simulink model "check_fence"  (Simulink 7.4)
settings: Solver=ode45  StartTime=0.0  StopTime=10.0  RelTol=1e-3
libraries: xbsIndex_r4 x293
(part 2 of 2)

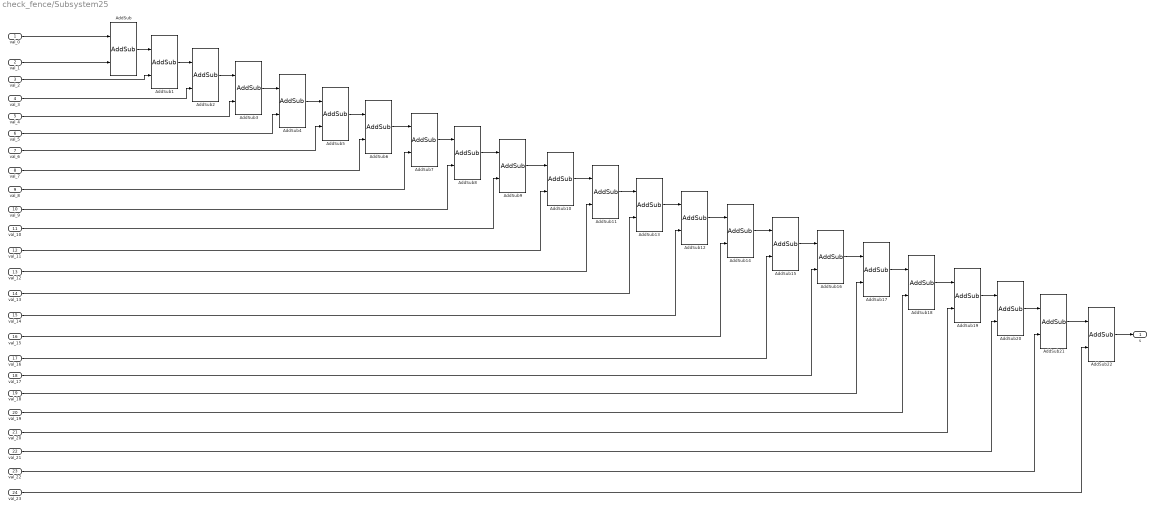
== system check_fence/Subsystem25 ==
  val_0 : Inport
  val_1 : Inport  Port=2
  val_2 : Inport  Port=3
  val_3 : Inport  Port=4
  val_4 : Inport  Port=5
  val_5 : Inport  Port=6
  val_6 : Inport  Port=7
  val_7 : Inport  Port=8
  val_8 : Inport  Port=9
  val_9 : Inport  Port=10
  val_10 : Inport  Port=11
  val_11 : Inport  Port=12
  val_12 : Inport  Port=13
  val_13 : Inport  Port=14
  val_14 : Inport  Port=15
  val_15 : Inport  Port=16
  val_16 : Inport  Port=17
  val_17 : Inport  Port=18
  val_18 : Inport  Port=19
  val_19 : Inport  Port=20
  val_20 : Inport  Port=21
  val_21 : Inport  Port=22
  val_22 : Inport  Port=23
  val_23 : Inport  Port=24
  AddSub{,1..22} (23 alike) : xbsIndex_r4/AddSub  mode=Addition  use_carryin=off  use_carryout=off  en=off  latency=0  precision=Full  arith_type=Unsigned  n_bits=16  bin_pt=14  quantization=Truncate  overflow=Wrap  dbl_ovrd=off  use_behavioral_HDL=off  hw_selection=Fabric  pipelined=off  block_type=addsub
  s : Outport
  wires:
  val_23/1 -> AddSub22/2
  val_22/1 -> AddSub21/2
  val_21/1 -> AddSub20/2
  val_20/1 -> AddSub19/2
  val_19/1 -> AddSub18/2
  val_18/1 -> AddSub17/2
  val_17/1 -> AddSub16/2
  val_16/1 -> AddSub15/2
  val_15/1 -> AddSub14/2
  val_14/1 -> AddSub12/2
  val_13/1 -> AddSub13/2
  val_12/1 -> AddSub11/2
  val_11/1 -> AddSub10/2
  val_10/1 -> AddSub9/2
  val_9/1 -> AddSub8/2
  val_8/1 -> AddSub7/2
  val_7/1 -> AddSub6/2
  val_6/1 -> AddSub5/2
  val_5/1 -> AddSub4/2
  val_4/1 -> AddSub3/2
  val_3/1 -> AddSub2/2
  val_2/1 -> AddSub1/2
  AddSub22/1 -> s/1
  AddSub21/1 -> AddSub22/1
  AddSub20/1 -> AddSub21/1
  AddSub19/1 -> AddSub20/1
  AddSub18/1 -> AddSub19/1
  AddSub17/1 -> AddSub18/1
  AddSub16/1 -> AddSub17/1
  AddSub15/1 -> AddSub16/1
  AddSub14/1 -> AddSub15/1
  AddSub12/1 -> AddSub14/1
  AddSub13/1 -> AddSub12/1
  AddSub11/1 -> AddSub13/1
  AddSub10/1 -> AddSub11/1
  AddSub9/1 -> AddSub10/1
  AddSub8/1 -> AddSub9/1
  AddSub7/1 -> AddSub8/1
  AddSub6/1 -> AddSub7/1
  AddSub5/1 -> AddSub6/1
  AddSub4/1 -> AddSub5/1
  AddSub3/1 -> AddSub4/1
  AddSub2/1 -> AddSub3/1
  AddSub1/1 -> AddSub2/1
  AddSub/1 -> AddSub1/1
  val_1/1 -> AddSub/2
  val_0/1 -> AddSub/1

== system check_fence/Subsystem3 ==
  warp_reg_addr : Inport
  warp_id : Inport  Port=2
  cta_id_in : Inport  Port=3
  cta_ld_en : Inport  Port=4
  is_fenced_in : Inport  Port=5
  is_fenced_ld_en : Inport  Port=6
  Constant : xbsIndex_r4/Constant  arith_type=Boolean  const=0  n_bits=16  bin_pt=14  explicit_period=off  period=1  equ=P=C  opselect=C  inp2=PCIN>>17  opr=+  inp1=P  carry=CIN  dbl_ovrd=off  block_type=constant
  Constant1 : xbsIndex_r4/Constant  arith_type=Boolean  const=0  n_bits=16  bin_pt=14  explicit_period=off  period=1  equ=P=C  opselect=C  inp2=PCIN>>17  opr=+  inp1=P  carry=CIN  dbl_ovrd=off  block_type=constant
  Constant2 : xbsIndex_r4/Constant  arith_type=Unsigned  const=0  n_bits=1  bin_pt=0  explicit_period=off  period=1  equ=P=C  opselect=C  inp2=PCIN>>17  opr=+  inp1=P  carry=CIN  dbl_ovrd=off  block_type=constant
  Mux : xbsIndex_r4/Mux  inputs=2  en=off  latency=0  precision=Full  arith_type=Unsigned  n_bits=16  bin_pt=14  quantization=Truncate  overflow=Wrap  dbl_ovrd=off  block_type=mux
  Mux1 : xbsIndex_r4/Mux  inputs=2  en=off  latency=0  precision=Full  arith_type=Unsigned  n_bits=16  bin_pt=14  quantization=Truncate  overflow=Wrap  dbl_ovrd=off  block_type=mux
  Mux2 : xbsIndex_r4/Mux  inputs=2  en=off  latency=0  precision=Full  arith_type=Unsigned  n_bits=16  bin_pt=14  quantization=Truncate  overflow=Wrap  dbl_ovrd=off  block_type=mux
  Register : xbsIndex_r4/Register  init=0  rst=off  en=on  dbl_ovrd=off  block_type=register
  Register1 : xbsIndex_r4/Register  init=0  rst=off  en=on  dbl_ovrd=off  block_type=register
  Relational : xbsIndex_r4/Relational  mode=a=b  en=off  latency=0  dbl_ovrd=off  block_type=relational
  Relational1 : xbsIndex_r4/Relational  mode=a=b  en=off  latency=0  dbl_ovrd=off  block_type=relational
  is_fenced_out : Outport
  data_valid : Outport  Port=2
  wires:
  cta_id_in/1 -> Register/1, Relational1/1
  is_fenced_in/1 -> Register1/1
  warp_reg_addr/1 -> Relational/1
  warp_id/1 -> Relational/2
  Mux/1 -> Register/2
  cta_ld_en/1 -> Mux/3
  Constant/1 -> Mux/2
  Relational/1 -> Mux/1, Mux1/1
  Mux1/1 -> Register1/2
  is_fenced_ld_en/1 -> Mux1/3
  Constant1/1 -> Mux1/2
  Relational1/1 -> Mux2/1, data_valid/1
  Constant2/1 -> Mux2/2
  Register/1 -> Relational1/2
  Register1/1 -> Mux2/3
  Mux2/1 -> is_fenced_out/1

== system check_fence/Subsystem4 ==
  warp_reg_addr : Inport
  warp_id : Inport  Port=2
  cta_id_in : Inport  Port=3
  cta_ld_en : Inport  Port=4
  is_fenced_in : Inport  Port=5
  is_fenced_ld_en : Inport  Port=6
  Constant : xbsIndex_r4/Constant  arith_type=Boolean  const=0  n_bits=16  bin_pt=14  explicit_period=off  period=1  equ=P=C  opselect=C  inp2=PCIN>>17  opr=+  inp1=P  carry=CIN  dbl_ovrd=off  block_type=constant
  Constant1 : xbsIndex_r4/Constant  arith_type=Boolean  const=0  n_bits=16  bin_pt=14  explicit_period=off  period=1  equ=P=C  opselect=C  inp2=PCIN>>17  opr=+  inp1=P  carry=CIN  dbl_ovrd=off  block_type=constant
  Constant2 : xbsIndex_r4/Constant  arith_type=Unsigned  const=0  n_bits=1  bin_pt=0  explicit_period=off  period=1  equ=P=C  opselect=C  inp2=PCIN>>17  opr=+  inp1=P  carry=CIN  dbl_ovrd=off  block_type=constant
  Mux : xbsIndex_r4/Mux  inputs=2  en=off  latency=0  precision=Full  arith_type=Unsigned  n_bits=16  bin_pt=14  quantization=Truncate  overflow=Wrap  dbl_ovrd=off  block_type=mux
  Mux1 : xbsIndex_r4/Mux  inputs=2  en=off  latency=0  precision=Full  arith_type=Unsigned  n_bits=16  bin_pt=14  quantization=Truncate  overflow=Wrap  dbl_ovrd=off  block_type=mux
  Mux2 : xbsIndex_r4/Mux  inputs=2  en=off  latency=0  precision=Full  arith_type=Unsigned  n_bits=16  bin_pt=14  quantization=Truncate  overflow=Wrap  dbl_ovrd=off  block_type=mux
  Register : xbsIndex_r4/Register  init=0  rst=off  en=on  dbl_ovrd=off  block_type=register
  Register1 : xbsIndex_r4/Register  init=0  rst=off  en=on  dbl_ovrd=off  block_type=register
  Relational : xbsIndex_r4/Relational  mode=a=b  en=off  latency=0  dbl_ovrd=off  block_type=relational
  Relational1 : xbsIndex_r4/Relational  mode=a=b  en=off  latency=0  dbl_ovrd=off  block_type=relational
  is_fenced_out : Outport
  data_valid : Outport  Port=2
  wires:
  Mux2/1 -> is_fenced_out/1
  Register1/1 -> Mux2/3
  Register/1 -> Relational1/2
  Constant2/1 -> Mux2/2
  Relational1/1 -> data_valid/1, Mux2/1
  Constant1/1 -> Mux1/2
  is_fenced_ld_en/1 -> Mux1/3
  Mux1/1 -> Register1/2
  Relational/1 -> Mux1/1, Mux/1
  Constant/1 -> Mux/2
  cta_ld_en/1 -> Mux/3
  Mux/1 -> Register/2
  warp_id/1 -> Relational/2
  warp_reg_addr/1 -> Relational/1
  is_fenced_in/1 -> Register1/1
  cta_id_in/1 -> Relational1/1, Register/1

== system check_fence/Subsystem5 ==
  warp_reg_addr : Inport
  warp_id : Inport  Port=2
  cta_id_in : Inport  Port=3
  cta_ld_en : Inport  Port=4
  is_fenced_in : Inport  Port=5
  is_fenced_ld_en : Inport  Port=6
  Constant : xbsIndex_r4/Constant  arith_type=Boolean  const=0  n_bits=16  bin_pt=14  explicit_period=off  period=1  equ=P=C  opselect=C  inp2=PCIN>>17  opr=+  inp1=P  carry=CIN  dbl_ovrd=off  block_type=constant
  Constant1 : xbsIndex_r4/Constant  arith_type=Boolean  const=0  n_bits=16  bin_pt=14  explicit_period=off  period=1  equ=P=C  opselect=C  inp2=PCIN>>17  opr=+  inp1=P  carry=CIN  dbl_ovrd=off  block_type=constant
  Constant2 : xbsIndex_r4/Constant  arith_type=Unsigned  const=0  n_bits=1  bin_pt=0  explicit_period=off  period=1  equ=P=C  opselect=C  inp2=PCIN>>17  opr=+  inp1=P  carry=CIN  dbl_ovrd=off  block_type=constant
  Mux : xbsIndex_r4/Mux  inputs=2  en=off  latency=0  precision=Full  arith_type=Unsigned  n_bits=16  bin_pt=14  quantization=Truncate  overflow=Wrap  dbl_ovrd=off  block_type=mux
  Mux1 : xbsIndex_r4/Mux  inputs=2  en=off  latency=0  precision=Full  arith_type=Unsigned  n_bits=16  bin_pt=14  quantization=Truncate  overflow=Wrap  dbl_ovrd=off  block_type=mux
  Mux2 : xbsIndex_r4/Mux  inputs=2  en=off  latency=0  precision=Full  arith_type=Unsigned  n_bits=16  bin_pt=14  quantization=Truncate  overflow=Wrap  dbl_ovrd=off  block_type=mux
  Register : xbsIndex_r4/Register  init=0  rst=off  en=on  dbl_ovrd=off  block_type=register
  Register1 : xbsIndex_r4/Register  init=0  rst=off  en=on  dbl_ovrd=off  block_type=register
  Relational : xbsIndex_r4/Relational  mode=a=b  en=off  latency=0  dbl_ovrd=off  block_type=relational
  Relational1 : xbsIndex_r4/Relational  mode=a=b  en=off  latency=0  dbl_ovrd=off  block_type=relational
  is_fenced_out : Outport
  data_valid : Outport  Port=2
  wires:
  cta_id_in/1 -> Register/1, Relational1/1
  is_fenced_in/1 -> Register1/1
  warp_reg_addr/1 -> Relational/1
  warp_id/1 -> Relational/2
  Mux/1 -> Register/2
  cta_ld_en/1 -> Mux/3
  Constant/1 -> Mux/2
  Relational/1 -> Mux/1, Mux1/1
  Mux1/1 -> Register1/2
  is_fenced_ld_en/1 -> Mux1/3
  Constant1/1 -> Mux1/2
  Relational1/1 -> Mux2/1, data_valid/1
  Constant2/1 -> Mux2/2
  Register/1 -> Relational1/2
  Register1/1 -> Mux2/3
  Mux2/1 -> is_fenced_out/1

== system check_fence/Subsystem6 ==
  warp_reg_addr : Inport
  warp_id : Inport  Port=2
  cta_id_in : Inport  Port=3
  cta_ld_en : Inport  Port=4
  is_fenced_in : Inport  Port=5
  is_fenced_ld_en : Inport  Port=6
  Constant : xbsIndex_r4/Constant  arith_type=Boolean  const=0  n_bits=16  bin_pt=14  explicit_period=off  period=1  equ=P=C  opselect=C  inp2=PCIN>>17  opr=+  inp1=P  carry=CIN  dbl_ovrd=off  block_type=constant
  Constant1 : xbsIndex_r4/Constant  arith_type=Boolean  const=0  n_bits=16  bin_pt=14  explicit_period=off  period=1  equ=P=C  opselect=C  inp2=PCIN>>17  opr=+  inp1=P  carry=CIN  dbl_ovrd=off  block_type=constant
  Constant2 : xbsIndex_r4/Constant  arith_type=Unsigned  const=0  n_bits=1  bin_pt=0  explicit_period=off  period=1  equ=P=C  opselect=C  inp2=PCIN>>17  opr=+  inp1=P  carry=CIN  dbl_ovrd=off  block_type=constant
  Mux : xbsIndex_r4/Mux  inputs=2  en=off  latency=0  precision=Full  arith_type=Unsigned  n_bits=16  bin_pt=14  quantization=Truncate  overflow=Wrap  dbl_ovrd=off  block_type=mux
  Mux1 : xbsIndex_r4/Mux  inputs=2  en=off  latency=0  precision=Full  arith_type=Unsigned  n_bits=16  bin_pt=14  quantization=Truncate  overflow=Wrap  dbl_ovrd=off  block_type=mux
  Mux2 : xbsIndex_r4/Mux  inputs=2  en=off  latency=0  precision=Full  arith_type=Unsigned  n_bits=16  bin_pt=14  quantization=Truncate  overflow=Wrap  dbl_ovrd=off  block_type=mux
  Register : xbsIndex_r4/Register  init=0  rst=off  en=on  dbl_ovrd=off  block_type=register
  Register1 : xbsIndex_r4/Register  init=0  rst=off  en=on  dbl_ovrd=off  block_type=register
  Relational : xbsIndex_r4/Relational  mode=a=b  en=off  latency=0  dbl_ovrd=off  block_type=relational
  Relational1 : xbsIndex_r4/Relational  mode=a=b  en=off  latency=0  dbl_ovrd=off  block_type=relational
  is_fenced_out : Outport
  data_valid : Outport  Port=2
  wires:
  Mux2/1 -> is_fenced_out/1
  Register1/1 -> Mux2/3
  Register/1 -> Relational1/2
  Constant2/1 -> Mux2/2
  Relational1/1 -> data_valid/1, Mux2/1
  Constant1/1 -> Mux1/2
  is_fenced_ld_en/1 -> Mux1/3
  Mux1/1 -> Register1/2
  Relational/1 -> Mux1/1, Mux/1
  Constant/1 -> Mux/2
  cta_ld_en/1 -> Mux/3
  Mux/1 -> Register/2
  warp_id/1 -> Relational/2
  warp_reg_addr/1 -> Relational/1
  is_fenced_in/1 -> Register1/1
  cta_id_in/1 -> Relational1/1, Register/1

== system check_fence/Subsystem7 ==
  warp_reg_addr : Inport
  warp_id : Inport  Port=2
  cta_id_in : Inport  Port=3
  cta_ld_en : Inport  Port=4
  is_fenced_in : Inport  Port=5
  is_fenced_ld_en : Inport  Port=6
  Constant : xbsIndex_r4/Constant  arith_type=Boolean  const=0  n_bits=16  bin_pt=14  explicit_period=off  period=1  equ=P=C  opselect=C  inp2=PCIN>>17  opr=+  inp1=P  carry=CIN  dbl_ovrd=off  block_type=constant
  Constant1 : xbsIndex_r4/Constant  arith_type=Boolean  const=0  n_bits=16  bin_pt=14  explicit_period=off  period=1  equ=P=C  opselect=C  inp2=PCIN>>17  opr=+  inp1=P  carry=CIN  dbl_ovrd=off  block_type=constant
  Constant2 : xbsIndex_r4/Constant  arith_type=Unsigned  const=0  n_bits=1  bin_pt=0  explicit_period=off  period=1  equ=P=C  opselect=C  inp2=PCIN>>17  opr=+  inp1=P  carry=CIN  dbl_ovrd=off  block_type=constant
  Mux : xbsIndex_r4/Mux  inputs=2  en=off  latency=0  precision=Full  arith_type=Unsigned  n_bits=16  bin_pt=14  quantization=Truncate  overflow=Wrap  dbl_ovrd=off  block_type=mux
  Mux1 : xbsIndex_r4/Mux  inputs=2  en=off  latency=0  precision=Full  arith_type=Unsigned  n_bits=16  bin_pt=14  quantization=Truncate  overflow=Wrap  dbl_ovrd=off  block_type=mux
  Mux2 : xbsIndex_r4/Mux  inputs=2  en=off  latency=0  precision=Full  arith_type=Unsigned  n_bits=16  bin_pt=14  quantization=Truncate  overflow=Wrap  dbl_ovrd=off  block_type=mux
  Register : xbsIndex_r4/Register  init=0  rst=off  en=on  dbl_ovrd=off  block_type=register
  Register1 : xbsIndex_r4/Register  init=0  rst=off  en=on  dbl_ovrd=off  block_type=register
  Relational : xbsIndex_r4/Relational  mode=a=b  en=off  latency=0  dbl_ovrd=off  block_type=relational
  Relational1 : xbsIndex_r4/Relational  mode=a=b  en=off  latency=0  dbl_ovrd=off  block_type=relational
  is_fenced_out : Outport
  data_valid : Outport  Port=2
  wires:
  Mux2/1 -> is_fenced_out/1
  Register1/1 -> Mux2/3
  Register/1 -> Relational1/2
  Constant2/1 -> Mux2/2
  Relational1/1 -> data_valid/1, Mux2/1
  Constant1/1 -> Mux1/2
  is_fenced_ld_en/1 -> Mux1/3
  Mux1/1 -> Register1/2
  Relational/1 -> Mux1/1, Mux/1
  Constant/1 -> Mux/2
  cta_ld_en/1 -> Mux/3
  Mux/1 -> Register/2
  warp_id/1 -> Relational/2
  warp_reg_addr/1 -> Relational/1
  is_fenced_in/1 -> Register1/1
  cta_id_in/1 -> Relational1/1, Register/1

== system check_fence/Subsystem8 ==
  warp_reg_addr : Inport
  warp_id : Inport  Port=2
  cta_id_in : Inport  Port=3
  cta_ld_en : Inport  Port=4
  is_fenced_in : Inport  Port=5
  is_fenced_ld_en : Inport  Port=6
  Constant : xbsIndex_r4/Constant  arith_type=Boolean  const=0  n_bits=16  bin_pt=14  explicit_period=off  period=1  equ=P=C  opselect=C  inp2=PCIN>>17  opr=+  inp1=P  carry=CIN  dbl_ovrd=off  block_type=constant
  Constant1 : xbsIndex_r4/Constant  arith_type=Boolean  const=0  n_bits=16  bin_pt=14  explicit_period=off  period=1  equ=P=C  opselect=C  inp2=PCIN>>17  opr=+  inp1=P  carry=CIN  dbl_ovrd=off  block_type=constant
  Constant2 : xbsIndex_r4/Constant  arith_type=Unsigned  const=0  n_bits=1  bin_pt=0  explicit_period=off  period=1  equ=P=C  opselect=C  inp2=PCIN>>17  opr=+  inp1=P  carry=CIN  dbl_ovrd=off  block_type=constant
  Mux : xbsIndex_r4/Mux  inputs=2  en=off  latency=0  precision=Full  arith_type=Unsigned  n_bits=16  bin_pt=14  quantization=Truncate  overflow=Wrap  dbl_ovrd=off  block_type=mux
  Mux1 : xbsIndex_r4/Mux  inputs=2  en=off  latency=0  precision=Full  arith_type=Unsigned  n_bits=16  bin_pt=14  quantization=Truncate  overflow=Wrap  dbl_ovrd=off  block_type=mux
  Mux2 : xbsIndex_r4/Mux  inputs=2  en=off  latency=0  precision=Full  arith_type=Unsigned  n_bits=16  bin_pt=14  quantization=Truncate  overflow=Wrap  dbl_ovrd=off  block_type=mux
  Register : xbsIndex_r4/Register  init=0  rst=off  en=on  dbl_ovrd=off  block_type=register
  Register1 : xbsIndex_r4/Register  init=0  rst=off  en=on  dbl_ovrd=off  block_type=register
  Relational : xbsIndex_r4/Relational  mode=a=b  en=off  latency=0  dbl_ovrd=off  block_type=relational
  Relational1 : xbsIndex_r4/Relational  mode=a=b  en=off  latency=0  dbl_ovrd=off  block_type=relational
  is_fenced_out : Outport
  data_valid : Outport  Port=2
  wires:
  cta_id_in/1 -> Register/1, Relational1/1
  is_fenced_in/1 -> Register1/1
  warp_reg_addr/1 -> Relational/1
  warp_id/1 -> Relational/2
  Mux/1 -> Register/2
  cta_ld_en/1 -> Mux/3
  Constant/1 -> Mux/2
  Relational/1 -> Mux/1, Mux1/1
  Mux1/1 -> Register1/2
  is_fenced_ld_en/1 -> Mux1/3
  Constant1/1 -> Mux1/2
  Relational1/1 -> Mux2/1, data_valid/1
  Constant2/1 -> Mux2/2
  Register/1 -> Relational1/2
  Register1/1 -> Mux2/3
  Mux2/1 -> is_fenced_out/1

== system check_fence/Subsystem9 ==
  warp_reg_addr : Inport
  warp_id : Inport  Port=2
  cta_id_in : Inport  Port=3
  cta_ld_en : Inport  Port=4
  is_fenced_in : Inport  Port=5
  is_fenced_ld_en : Inport  Port=6
  Constant : xbsIndex_r4/Constant  arith_type=Boolean  const=0  n_bits=16  bin_pt=14  explicit_period=off  period=1  equ=P=C  opselect=C  inp2=PCIN>>17  opr=+  inp1=P  carry=CIN  dbl_ovrd=off  block_type=constant
  Constant1 : xbsIndex_r4/Constant  arith_type=Boolean  const=0  n_bits=16  bin_pt=14  explicit_period=off  period=1  equ=P=C  opselect=C  inp2=PCIN>>17  opr=+  inp1=P  carry=CIN  dbl_ovrd=off  block_type=constant
  Constant2 : xbsIndex_r4/Constant  arith_type=Unsigned  const=0  n_bits=1  bin_pt=0  explicit_period=off  period=1  equ=P=C  opselect=C  inp2=PCIN>>17  opr=+  inp1=P  carry=CIN  dbl_ovrd=off  block_type=constant
  Mux : xbsIndex_r4/Mux  inputs=2  en=off  latency=0  precision=Full  arith_type=Unsigned  n_bits=16  bin_pt=14  quantization=Truncate  overflow=Wrap  dbl_ovrd=off  block_type=mux
  Mux1 : xbsIndex_r4/Mux  inputs=2  en=off  latency=0  precision=Full  arith_type=Unsigned  n_bits=16  bin_pt=14  quantization=Truncate  overflow=Wrap  dbl_ovrd=off  block_type=mux
  Mux2 : xbsIndex_r4/Mux  inputs=2  en=off  latency=0  precision=Full  arith_type=Unsigned  n_bits=16  bin_pt=14  quantization=Truncate  overflow=Wrap  dbl_ovrd=off  block_type=mux
  Register : xbsIndex_r4/Register  init=0  rst=off  en=on  dbl_ovrd=off  block_type=register
  Register1 : xbsIndex_r4/Register  init=0  rst=off  en=on  dbl_ovrd=off  block_type=register
  Relational : xbsIndex_r4/Relational  mode=a=b  en=off  latency=0  dbl_ovrd=off  block_type=relational
  Relational1 : xbsIndex_r4/Relational  mode=a=b  en=off  latency=0  dbl_ovrd=off  block_type=relational
  is_fenced_out : Outport
  data_valid : Outport  Port=2
  wires:
  Mux2/1 -> is_fenced_out/1
  Register1/1 -> Mux2/3
  Register/1 -> Relational1/2
  Constant2/1 -> Mux2/2
  Relational1/1 -> data_valid/1, Mux2/1
  Constant1/1 -> Mux1/2
  is_fenced_ld_en/1 -> Mux1/3
  Mux1/1 -> Register1/2
  Relational/1 -> Mux1/1, Mux/1
  Constant/1 -> Mux/2
  cta_ld_en/1 -> Mux/3
  Mux/1 -> Register/2
  warp_id/1 -> Relational/2
  warp_reg_addr/1 -> Relational/1
  is_fenced_in/1 -> Register1/1
  cta_id_in/1 -> Relational1/1, Register/1
